simulink model "ampc_pH_linearization"  (R2021a)
settings: Solver=ode45  StartTime=0.0  StopTime=400  MaxStep=0.3  RelTol=1e-3
undefined symbols (not defined in the file or in its folder): sigbuilder_block
libraries: mpclib x1, simulink x1
settings Model: Creator=NIFEMI  LastModifiedBy=USER
settings SolverCC: ZeroCrossAlgorithm=Adaptive  AlgebraicLoopSolver=LineSearch
settings DataIOCC: ReturnWorkspaceOutputs=off
settings DebuggingCC: PregeneratedLibrarySubsystemCodeDiagnostic=none  SFMachineParentedDataDiag=warning  ArithmeticOperatorsInVariantConditions=warning
settings SFSimCC: CustomCodeUndefinedFunction=UseInterfaceOnly

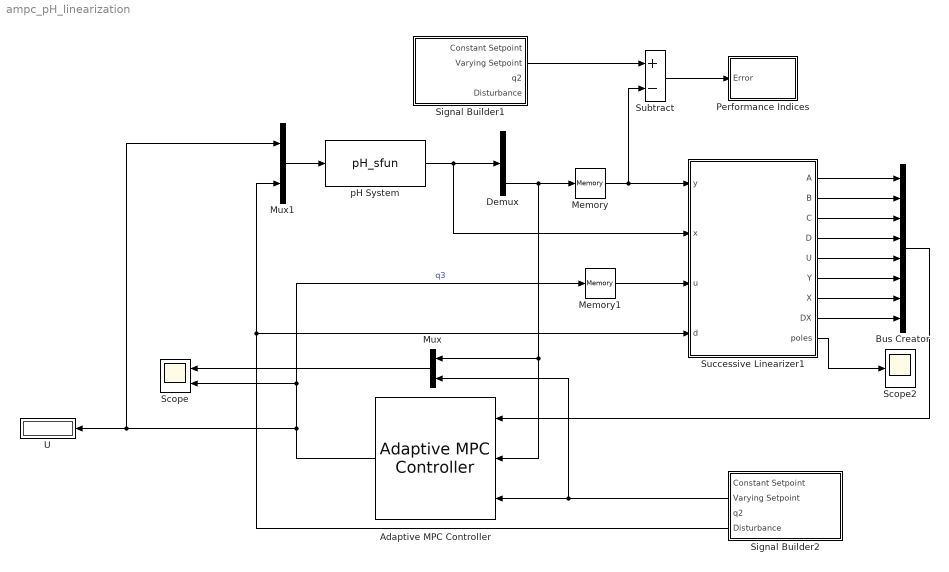
== system ampc_pH_linearization ==
  Adaptive MPC Controller : mpclib/Adaptive MPC Controller  SCDEnableBlockLinearizationSpecification=on  mpcobj=mpcobj_L  enable_value=0  updateMPCinCallerWorkspace=on  md_inport=off  mv_inport=off  uref_inport=off  return_cost=off  return_mvseq=off  return_qpstatus=off  return_xseq=off  return_state=off  return_ovseq=off  state_inport=off  isltv_plant=off  umin_inport=off  umax_inport=off  ymin_inport=off  ymax_inport=off  cc_inport=off  ywt_inport=off  uwt_inport=off  duwt_inport=off  rhoeps_inport=off  pm_inport=off  MaximumP=10  HorizonChoice=FixedHorizon  BlockDataType=double  SampleTimeInherited=off  switch_inport=off
  Bus Creator : BusCreator  Inputs=8
  Demux : Demux  Outputs=3
  Memory : Memory  InitialCondition=7
  Memory1 : Memory  InitialCondition=15.6
  Mux : Mux  Inputs=2
  Mux1 : Mux  Inputs=2
  Performance Indices : Subsystem
  Scope : Scope  NumInputPorts=2
  Scope2 : Scope
  Signal Builder1 : Subsystem  Tag=STV Subsys  LoadFcn=sigbuilder_block('load');  StartFcn=sigbuilder_block('start');  StopFcn=sigbuilder_block('stop');  ClipboardFcn=sigbuilder_block('clipboard');  mask(Sigbuilder block){tuvar=[0:10]}
      mask help: Simulink:masks:SigbuilderBlock_MD
      mask init:
      | if ~strcmp(get_param(bdroot(gcbh),'SimulationStatus'),'stopped') tuvar = sigbuilder_block('maskInit'); end
      settings: CopyFcn=sigbuilder_block('copy');  DeleteFcn=sigbuilder_block('delete');  ModelCloseFcn=sigbuilder_block('modelClose');  PreSaveFcn=sigbuilder_block('preSave');  PauseFcn=sigbuilder_block('pause');  ContinueFcn=sigbuilder_block('continue');  NameChangeFcn=sigbuilder_block('namechange');  OpenFcn=sigbuilder_block('open',[301 130.5 653.5 349.5 ]);  CloseFcn=sigbuilder_block('close');
      mask Display: plot(0, 0, 100, 100,[2, 2, 32, 32, 2], [68, 8, 8, 68, 68],[32, 2], [38, 38], [32, 19, 2],[53, 60, 44], [32, 17, 17, 2],[16, 16, 31, 31]);txt = getActiveGroup(gcbh);text(2, 100, txt,'verticalAlignment', 'top');
  Signal Builder2 : Subsystem  Tag=STV Subsys  LoadFcn=sigbuilder_block('load');  StartFcn=sigbuilder_block('start');  StopFcn=sigbuilder_block('stop');  ClipboardFcn=sigbuilder_block('clipboard');  mask(Sigbuilder block){tuvar=[0:10]}
      mask help: Simulink:masks:SigbuilderBlock_MD
      mask init:
      | if ~strcmp(get_param(bdroot(gcbh),'SimulationStatus'),'stopped') tuvar = sigbuilder_block('maskInit'); end
      settings: CopyFcn=sigbuilder_block('copy');  DeleteFcn=sigbuilder_block('delete');  ModelCloseFcn=sigbuilder_block('modelClose');  PreSaveFcn=sigbuilder_block('preSave');  PauseFcn=sigbuilder_block('pause');  ContinueFcn=sigbuilder_block('continue');  NameChangeFcn=sigbuilder_block('namechange');  OpenFcn=sigbuilder_block('open',[301 130.5 653.5 349.5 ]);  CloseFcn=sigbuilder_block('close');
      mask Display: plot(0, 0, 100, 100,[2, 2, 32, 32, 2], [68, 8, 8, 68, 68],[32, 2], [38, 38], [32, 19, 2],[53, 60, 44], [32, 17, 17, 2],[16, 16, 31, 31]);txt = getActiveGroup(gcbh);text(2, 100, txt,'verticalAlignment', 'top');
  Subtract : Sum  Inputs=+-
  Successive Linearizer1 : MATLAB Function  TreatAsAtomicUnit=on  SystemSampleTime=0.5
  U : Display
  pH System : S-Function  FunctionName=pH_sfun  SFunctionDeploymentMode=off  EnableBusSupport=off
  wires:
  Successive Linearizer1/1(A) -> Bus Creator/1
  Successive Linearizer1/2(B) -> Bus Creator/2
  Successive Linearizer1/3(C) -> Bus Creator/3
  Successive Linearizer1/5(U) -> Bus Creator/5
  Successive Linearizer1/6(Y) -> Bus Creator/6
  Successive Linearizer1/7(X) -> Bus Creator/7
  Successive Linearizer1/8(DX) -> Bus Creator/8
  Successive Linearizer1/4(D) -> Bus Creator/4
  Bus Creator/1 -> Adaptive MPC Controller/1
  Mux/1 -> Scope/1
  Subtract/1 -> Performance Indices/1(Error)
  Signal Builder2/2(Varying Setpoint) -> Mux/2, Adaptive MPC Controller/3
  Adaptive MPC Controller/1 -> Memory1/1, Scope/2, Mux1/1, U/1  "q3"
  Memory/1 -> Subtract/2, Successive Linearizer1/1(y)
  Successive Linearizer1/9(poles) -> Scope2/1
  Demux/3 -> Adaptive MPC Controller/2, Mux/1, Memory/1
  pH System/1 -> Successive Linearizer1/2(x), Demux/1
  Mux1/1 -> pH System/1
  Signal Builder2/4(Disturbance) -> Successive Linearizer1/4(d), Mux1/2
  Signal Builder1/2(Varying Setpoint) -> Subtract/1
  Memory1/1 -> Successive Linearizer1/3(u)

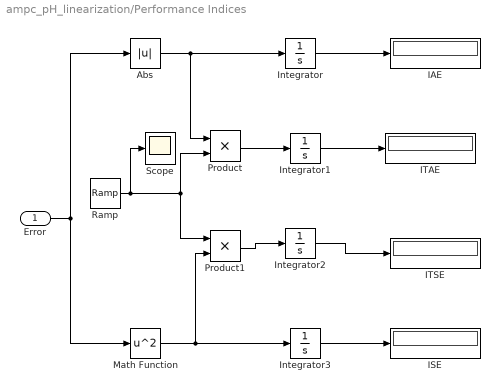
== system ampc_pH_linearization/Performance Indices ==
  Error : Inport
  Abs : Abs
  IAE : Display
  ISE : Display
  ITAE : Display
  ITSE : Display
  Integrator{,1..3} (4 alike) : Integrator
  Math Function : Math  Operator=square  SignedPower=on  SaturateOnIntegerOverflow=on
  Product : Product  RndMeth=Zero
  Product1 : Product  RndMeth=Zero
  Ramp : simulink/Sources/Ramp  slope=1  start=0  InitialOutput=0
  Scope : Scope
  wires:
  Error/1 -> Math Function/1, Abs/1
  Abs/1 -> Integrator/1, Product/1
  Integrator/1 -> IAE/1
  Ramp/1 -> Product/2, Product1/1, Scope/1
  Math Function/1 -> Integrator3/1, Product1/2
  Product1/1 -> Integrator2/1
  Product/1 -> Integrator1/1
  Integrator3/1 -> ISE/1
  Integrator2/1 -> ITSE/1
  Integrator1/1 -> ITAE/1

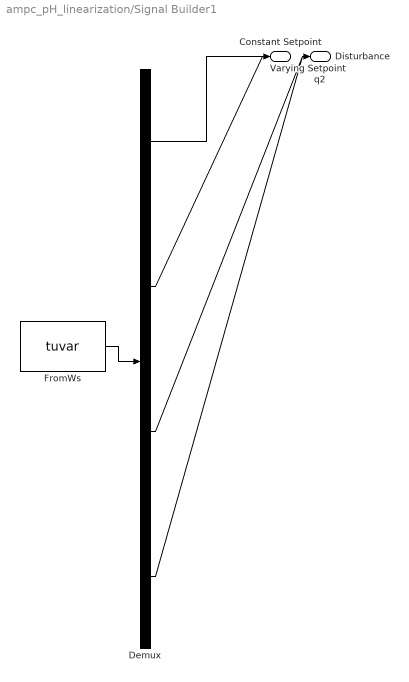
== system ampc_pH_linearization/Signal Builder1 ==
  Demux : Demux  Tag=STV Demux
      settings: DisplayOption=none
  FromWs : FromWorkspace  Tag=STV FromWs  VariableName=tuvar
      SigBuilderData=|
      | common.afterFinalStr = 'Extrapolate'
      | common.sampleTime = 0
      | dataSet(1).timeRange = [0 400]
      | dataSet(1).name = 'Servo'
      | dataSet(2).timeRange = [0 400]
      | dataSet(2).name = 'Regulatory'
      | sbobj.Groups(1).Name = 'Servo'
      | sbobj.Groups(1).Signals(1).Name = 'Constant Setpoint'
      | sbobj.Groups(1).Signals(1).XData = [0 400]
      | sbobj.Groups(1).Signals(1).YData = [7 7]
      | sbobj.Groups(1).Signals(2).Name = 'Varying Setpoint'
      | sbobj.Groups(1).Signals(2).XData = [0 50 50 200 200 300 300 400]
      | sbobj.Groups(1).Signals(2).YData = [7 7 5 5 10 10 7 7]
      | sbobj.Groups(1).Signals(3).Name = 'q2'
      | sbobj.Groups(1).Signals(3).XData = [0 400]
      | sbobj.Groups(1).Signals(3).YData = [0.55 0.55]
      | sbobj.Groups(1).Signals(4).Name = 'Disturbance'
      | sbobj.Groups(1).Signals(4).XData = [0 100 100 200 200 300 300 400]
      | sbobj.Groups(1).Signals(4).YData = [0.55 0.55 1.5 1.5 0.05 0.05 0.55 0.55]
      | sbobj.Groups(1).TimeRange = [0 400]
      | sbobj.Groups(2).Name = 'Regulatory'
      | sbobj.Groups(2).Signals(1).Name = 'Constant Setpoint'
      | sbobj.Groups(2).Signals(1).XData = [0 400]
      | sbobj.Groups(2).Signals(1).YData = [0 0]
      | sbobj.Groups(2).Signals(2).Name = 'Varying Setpoint'
      | sbobj.Groups(2).Signals(2).XData = [0 400]
      | sbobj.Groups(2).Signals(2).YData = [7 7]
      | sbobj.Groups(2).Signals(3).Name = 'q2'
      | sbobj.Groups(2).Signals(3).XData = [0 30 30 60 60 90 90 120 120 150 150 400]
      | sbobj.Groups(2).Signals(3).YData = [0.55 0.55 1.2 1.2 2 2 1 1 0 0 0.55 0.55]
      | sbobj.Groups(2).Signals(4).Name = 'Disturbance'
      | sbobj.Groups(2).Signals(4).XData = [0 400]
      | sbobj.Groups(2).Signals(4).YData = [0 0]
      | sbobj.Groups(2).TimeRange = [0 400]
  Constant Setpoint : Outport  Tag=STV Outport
  Varying Setpoint : Outport  Tag=STV Outport  Port=2  VectorParamsAs1DForOutWhenUnconnected=off
  q2 : Outport  Tag=STV Outport  Port=3  VectorParamsAs1DForOutWhenUnconnected=off
  Disturbance : Outport  Tag=STV Outport  Port=4
  wires:
  FromWs/1 -> Demux/1
  Demux/1 -> Constant Setpoint/1
  Demux/2 -> Varying Setpoint/1
  Demux/3 -> q2/1
  Demux/4 -> Disturbance/1

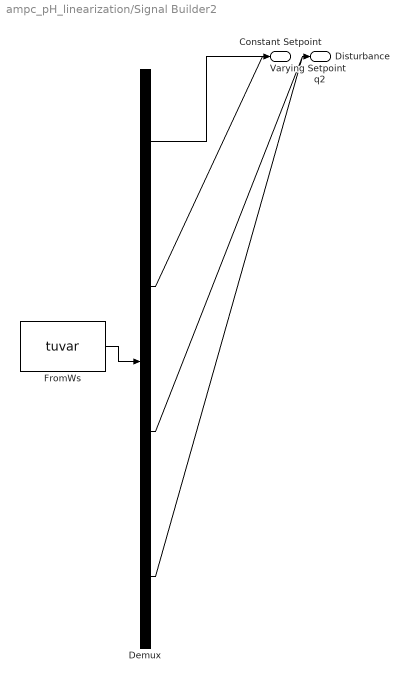
== system ampc_pH_linearization/Signal Builder2 ==
  Demux : Demux  Tag=STV Demux
      settings: DisplayOption=none
  FromWs : FromWorkspace  Tag=STV FromWs  VariableName=tuvar
      SigBuilderData=|
      | common.afterFinalStr = 'Extrapolate'
      | common.sampleTime = 0
      | dataSet(1).timeRange = [0 400]
      | dataSet(1).name = 'Servo'
      | dataSet(2).timeRange = [0 400]
      | dataSet(2).name = 'Regulatory'
      | sbobj.Groups(1).Name = 'Servo'
      | sbobj.Groups(1).Signals(1).Name = 'Constant Setpoint'
      | sbobj.Groups(1).Signals(1).XData = [0 400]
      | sbobj.Groups(1).Signals(1).YData = [7 7]
      | sbobj.Groups(1).Signals(2).Name = 'Varying Setpoint'
      | sbobj.Groups(1).Signals(2).XData = [0 50 50 200 200 300 300 400]
      | sbobj.Groups(1).Signals(2).YData = [7 7 5 5 10 10 7 7]
      | sbobj.Groups(1).Signals(3).Name = 'q2'
      | sbobj.Groups(1).Signals(3).XData = [0 400]
      | sbobj.Groups(1).Signals(3).YData = [0.55 0.55]
      | sbobj.Groups(1).Signals(4).Name = 'Disturbance'
      | sbobj.Groups(1).Signals(4).XData = [0 100 100 200 200 300 300 400]
      | sbobj.Groups(1).Signals(4).YData = [0.55 0.55 1.5 1.5 0.05 0.05 0.55 0.55]
      | sbobj.Groups(1).TimeRange = [0 400]
      | sbobj.Groups(2).Name = 'Regulatory'
      | sbobj.Groups(2).Signals(1).Name = 'Constant Setpoint'
      | sbobj.Groups(2).Signals(1).XData = [0 400]
      | sbobj.Groups(2).Signals(1).YData = [0 0]
      | sbobj.Groups(2).Signals(2).Name = 'Varying Setpoint'
      | sbobj.Groups(2).Signals(2).XData = [0 400]
      | sbobj.Groups(2).Signals(2).YData = [7 7]
      | sbobj.Groups(2).Signals(3).Name = 'q2'
      | sbobj.Groups(2).Signals(3).XData = [0 30 30 60 60 90 90 120 120 150 150 400]
      | sbobj.Groups(2).Signals(3).YData = [0.55 0.55 1.2 1.2 2 2 1 1 0 0 0.55 0.55]
      | sbobj.Groups(2).Signals(4).Name = 'Disturbance'
      | sbobj.Groups(2).Signals(4).XData = [0 400]
      | sbobj.Groups(2).Signals(4).YData = [0 0]
      | sbobj.Groups(2).TimeRange = [0 400]
  Constant Setpoint : Outport  Tag=STV Outport
  Varying Setpoint : Outport  Tag=STV Outport  Port=2  VectorParamsAs1DForOutWhenUnconnected=off
  q2 : Outport  Tag=STV Outport  Port=3  VectorParamsAs1DForOutWhenUnconnected=off
  Disturbance : Outport  Tag=STV Outport  Port=4
  wires:
  FromWs/1 -> Demux/1
  Demux/1 -> Constant Setpoint/1
  Demux/2 -> Varying Setpoint/1
  Demux/3 -> q2/1
  Demux/4 -> Disturbance/1

== matlab function ampc_pH_linearization/Successive Linearizer1 ==
  data: y input size=[1,1]; x input; A output size=[2,2]; B output size=[2 1]; C output size=[1,2]; D output size=[1 1]; U output size=[1,1]; Y output size=[1,1]; X output size=[2,1]; DX output size=[2,1]; u input; d input; poles output
function [A, B, C, D, U, Y, X, DX,poles] = fcn(y, x, u, d)

%%%%%%%%%%%%%%%%%%%%%%%%%%%%%%%%%%%%%%%%%%%%%%%%%%%%%%%
%#codegen

% Define constant outputs
Ts = 0.5;
U = u(1) ;
Y = y ;
X = x(1:2) ;



% Analytical linearization of mechanistic CSTR model (continuous time)
% [A, Bo] = getContinuous(T, CA, CAi, Ti, Tc);
[a, b, c, d] = getContinuous(y, x, u, d, Ts)  ;

% Convert continuous to discrete time
% [A, Bo] = getDiscrete(A, Bo, Ts);
[A, Bo, C, D] = getDiscrete(a, b, c, d, Ts)   ;
% Last column of B contains the constant offset contribution.
DX = Bo(:,2);
B = Bo(:,1);
% Compute poles
poles = abs(eig(A));

end

%%%%%%%%%%%%%%%%%%%%%%%%%%%%%%%%%%%%%%%%%%%%%%%%%%%%%
%%%%%%%%%%%%%%%%%%%%%%%%%%%%%%%%%%%

function [a, b, c, d] = getContinuous(y, x, u, d, Ts)




% [A, B, C, D] = get_discrete_model(y, x, u, d, Ts)   ;

%%%%%%%%%%%%%%%%%%%%%%%%%%%%%%%%%%%%%
    q3 = u(1);
    q2 = d(1);
    
    Wa4 = x(1);
    Wb4 = x(2);
    
    A = 207;
    h = 14;
    q1e = 16.6;
    Wa1 = 0.003;
    Wa2 = -0.03;
    Wa3 = -0.00305;
    Wb1 = 0;
    Wb2 = 0.03;
    Wb3 = 5e-5;
    pK1 = 6.35;
    pK2 = 10.25;
    dWa4dt = (1/(h*A))*((q1e*(Wa1 - Wa4)) + (q2*(Wa2 - Wa4)) + (q3*(Wa3 - Wa4)));
    dWb4dt = (1/(h*A))*((q1e*(Wb1 - Wb4)) + (q2*(Wb2 - Wb4)) + (q3*(Wb3 - Wb4)));
    dxdt = [dWa4dt; dWb4dt];

    %%%%%%%%%%%%%%%%%%%%%%%%%%%%%%%%%%
    q3 = u(1);
    q2 = d(1);
    
    Wa4 = x(1);
    Wb4 = x(2);

    pH = y(1);   
    
a = [ - q2/2898 - q3/2898 - 83/14490,  0;
         0, - q2/2898 - q3/2898 - 83/14490];
     
b = [- Wa4/2898 - 61/57960000 dWa4dt;
           1/57960000 - Wb4/2898 dWb4dt];
       
c = [-1/(log(10)/10^pH + 10^(pH - 14)*log(10) + (Wb4*(2*10^(pH - pK2) + 1)*(10^(pK1 - pH)*log(10) - 10^(pH - pK2)*log(10)))/(10^(pK1 - pH) + 10^(pH - pK2) + 1)^2 + (2*10^(pH - pK2)*Wb4*log(10))/(10^(pK1 - pH) + 10^(pH - pK2) + 1)),...
        -(2*10^(pH - pK2) + 1)/((10^(pK1 - pH) + 10^(pH - pK2) + 1)*(log(10)/10^pH + 10^(pH - 14)*log(10) + (Wb4*(2*10^(pH - pK2) + 1)*(10^(pK1 - pH)*log(10) - 10^(pH - pK2)*log(10)))/(10^(pK1 - pH) + 10^(pH - pK2) + 1)^2 + (2*10^(pH - pK2)*Wb4*log(10))/(10^(pK1 - pH) + 10^(pH - pK2) + 1)))
        ];
    
d = 0;

    
    
       
    
    %%%%%%%%%%%%%%%%%%%%%%%%%%%%%%
    
       

end


function [A, B, C, D] = getDiscrete(a, b,c,d, Ts)
% Convert to discrete time
A = expm(a*Ts);
nx = size(b,1);
n = 4;  % Number of points for Simpson's Rule, an even integer >= 2.
% Use Simpson's rule to compute integral(0,Ts){expm(a*s)*ds*b}
h = Ts/n;
Ai = eye(nx) + A;        % First and last terms;
Coef = 2;
for i = 1:n-1
    if Coef == 2
        Coef = 4;
    else
        Coef = 2;
    end
    Ai = Ai + Coef*expm(a*i*h);     % Intermediate terms
end
B = (h/3)*Ai*b;

C = c  ;
D = d ;

end
